simulink model "Roadsense_ScenarioAdapters"  (R2025b)
settings: Solver=FixedStepDiscrete  StartTime=0.0  StopTime=1.0  FixedStep=RsTsBase  RelTol=1e-3
undefined symbols (not defined in the file or in its folder): RsMaxDetections, RsMaxLidarPoints, RsMaxReferencePoints, RsTsBase, RsTsControl, RsTsFusion, RsTsLidarPerception, RsTsPlanning, RsTsSemanticInference
settings Model: DataDictionary=Roadsense_Data.sldd  Creator=ragur  LastModifiedBy=ragur

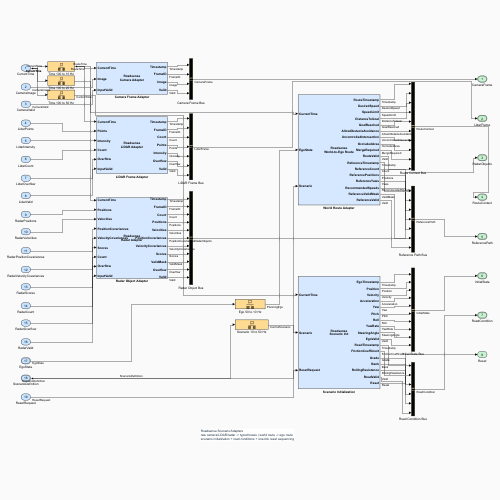
[thumbnail: Simulink's stored preview of the top-level diagram]
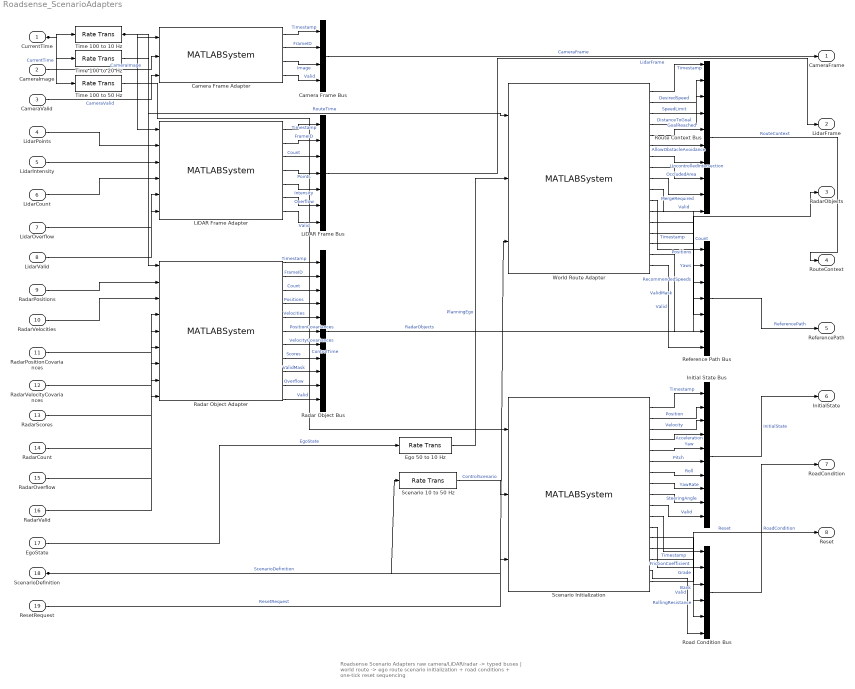
== system Roadsense_ScenarioAdapters ==
  note: Roadsense Scenario Adapters
      | raw camera/LiDAR/radar -> typed buses | world route -> ego route
      | scenario initialization + road conditions + one-tick reset sequencing
  CurrentTime : Inport  OutDataTypeStr=double  PortDimensions=1  SampleTime=RsTsBase
  CameraImage : Inport  Port=2  OutDataTypeStr=uint8  PortDimensions=[480 640 3]  SampleTime=RsTsSemanticInference
  CameraValid : Inport  Port=3  OutDataTypeStr=boolean  PortDimensions=1  SampleTime=RsTsSemanticInference
  LidarPoints : Inport  Port=4  OutDataTypeStr=single  PortDimensions=[120000 3]  SampleTime=RsTsLidarPerception
  LidarIntensity : Inport  Port=5  OutDataTypeStr=single  PortDimensions=[120000 1]  SampleTime=RsTsLidarPerception
  LidarCount : Inport  Port=6  OutDataTypeStr=uint32  PortDimensions=1  SampleTime=RsTsLidarPerception
  LidarOverflow : Inport  Port=7  OutDataTypeStr=boolean  PortDimensions=1  SampleTime=RsTsLidarPerception
  LidarValid : Inport  Port=8  OutDataTypeStr=boolean  PortDimensions=1  SampleTime=RsTsLidarPerception
  RadarPositions : Inport  Port=9  OutDataTypeStr=single  PortDimensions=[256 3]  SampleTime=RsTsFusion
  RadarVelocities : Inport  Port=10  OutDataTypeStr=single  PortDimensions=[256 3]  SampleTime=RsTsFusion
  RadarPositionCovariances : Inport  Port=11  OutDataTypeStr=single  PortDimensions=[3 3 256]  SampleTime=RsTsFusion
  RadarVelocityCovariances : Inport  Port=12  OutDataTypeStr=single  PortDimensions=[3 3 256]  SampleTime=RsTsFusion
  RadarScores : Inport  Port=13  OutDataTypeStr=single  PortDimensions=[256 1]  SampleTime=RsTsFusion
  RadarCount : Inport  Port=14  OutDataTypeStr=uint16  PortDimensions=1  SampleTime=RsTsFusion
  RadarOverflow : Inport  Port=15  OutDataTypeStr=boolean  PortDimensions=1  SampleTime=RsTsFusion
  RadarValid : Inport  Port=16  OutDataTypeStr=boolean  PortDimensions=1  SampleTime=RsTsFusion
  EgoState : Inport  Port=17  OutDataTypeStr=Bus: RsEgoStateBus  PortDimensions=1  SampleTime=RsTsControl
  ScenarioDefinition : Inport  Port=18  OutDataTypeStr=Bus: RsScenarioDefinitionBus  PortDimensions=1  SampleTime=RsTsPlanning
  ResetRequest : Inport  Port=19  OutDataTypeStr=boolean  PortDimensions=1  SampleTime=RsTsControl
  Camera Frame Adapter : MATLABSystem  System=RoadsenseCameraFrameAdapterSystem  SimulateUsing=Code generation
      mask Type: RoadsenseCameraFrameAdapterSystem
  Camera Frame Bus : BusCreator  Inputs=4  OutDataTypeStr=Bus: RsCameraFrameBus
  Ego 50 to 10 Hz : RateTransition  OutPortSampleTime=RsTsPlanning
  Initial State Bus : BusCreator  Inputs=10  OutDataTypeStr=Bus: RsEgoStateBus
  LiDAR Frame Adapter : MATLABSystem  System=RoadsenseLidarFrameAdapterSystem  MaxPoints=double(RsMaxLidarPoints)  SimulateUsing=Code generation
      mask Type: RoadsenseLidarFrameAdapterSystem
  LiDAR Frame Bus : BusCreator  Inputs=7  OutDataTypeStr=Bus: RsLidarFrameBus
  Radar Object Adapter : MATLABSystem  System=RoadsenseRadarObjectAdapterSystem  MaxDetections=double(RsMaxDetections)  SimulateUsing=Code generation
      mask Type: RoadsenseRadarObjectAdapterSystem
  Radar Object Bus : BusCreator  Inputs=11  OutDataTypeStr=Bus: RsRadarObjectListBus
  Reference Path Bus : BusCreator  Inputs=7  OutDataTypeStr=Bus: RsReferencePathBus
  Road Condition Bus : BusCreator  Inputs=6  OutDataTypeStr=Bus: RsRoadConditionBus
  Route Context Bus : BusCreator  Inputs=10  OutDataTypeStr=Bus: RsRouteContextBus
  Scenario 10 to 50 Hz : RateTransition  OutPortSampleTime=RsTsControl
  Scenario Initialization : MATLABSystem  System=RoadsenseScenarioInitializationSystem  SimulateUsing=Code generation
      mask Type: RoadsenseScenarioInitializationSystem
  Time 100 to 10 Hz : RateTransition  OutPortSampleTime=RsTsPlanning
  Time 100 to 20 Hz : RateTransition  OutPortSampleTime=RsTsFusion
  Time 100 to 50 Hz : RateTransition  OutPortSampleTime=RsTsControl
  World Route Adapter : MATLABSystem  System=RoadsenseRouteAdapterSystem  MaxReferencePoints=double(RsMaxReferencePoints)  SimulateUsing=Code generation
      mask Type: RoadsenseRouteAdapterSystem
  CameraFrame : Outport  OutDataTypeStr=Bus: RsCameraFrameBus
  LidarFrame : Outport  Port=2  OutDataTypeStr=Bus: RsLidarFrameBus
  RadarObjects : Outport  Port=3  OutDataTypeStr=Bus: RsRadarObjectListBus
  RouteContext : Outport  Port=4  OutDataTypeStr=Bus: RsRouteContextBus
  ReferencePath : Outport  Port=5  OutDataTypeStr=Bus: RsReferencePathBus
  InitialState : Outport  Port=6  OutDataTypeStr=Bus: RsEgoStateBus
  RoadCondition : Outport  Port=7  OutDataTypeStr=Bus: RsRoadConditionBus
  Reset : Outport  Port=8  OutDataTypeStr=boolean
  wires:
  CurrentTime/1 -> Time 100 to 10 Hz/1, Time 100 to 20 Hz/1, Time 100 to 50 Hz/1  "CurrentTime"
  EgoState/1 -> Ego 50 to 10 Hz/1  "EgoState"
  ScenarioDefinition/1 -> Scenario 10 to 50 Hz/1, World Route Adapter/3  "ScenarioDefinition"
  Time 100 to 10 Hz/1 -> Camera Frame Adapter/1, LiDAR Frame Adapter/1, World Route Adapter/1  "RouteTime"
  CameraImage/1 -> Camera Frame Adapter/2  "CameraImage"
  CameraValid/1 -> Camera Frame Adapter/3  "CameraValid"
  Camera Frame Adapter/1 -> Camera Frame Bus/1  "Timestamp"
  Camera Frame Adapter/2 -> Camera Frame Bus/2  "FrameID"
  Camera Frame Adapter/3 -> Camera Frame Bus/3  "Image"
  Camera Frame Adapter/4 -> Camera Frame Bus/4  "Valid"
  LidarPoints/1 -> LiDAR Frame Adapter/2
  LidarIntensity/1 -> LiDAR Frame Adapter/3
  LidarCount/1 -> LiDAR Frame Adapter/4
  LidarOverflow/1 -> LiDAR Frame Adapter/5
  LidarValid/1 -> LiDAR Frame Adapter/6
  LiDAR Frame Adapter/1 -> LiDAR Frame Bus/1  "Timestamp"
  LiDAR Frame Adapter/2 -> LiDAR Frame Bus/2  "FrameID"
  LiDAR Frame Adapter/3 -> LiDAR Frame Bus/3  "Count"
  LiDAR Frame Adapter/4 -> LiDAR Frame Bus/4  "Points"
  LiDAR Frame Adapter/5 -> LiDAR Frame Bus/5  "Intensity"
  LiDAR Frame Adapter/6 -> LiDAR Frame Bus/6  "Overflow"
  LiDAR Frame Adapter/7 -> LiDAR Frame Bus/7  "Valid"
  Time 100 to 20 Hz/1 -> Radar Object Adapter/1
  RadarPositions/1 -> Radar Object Adapter/2
  RadarVelocities/1 -> Radar Object Adapter/3
  RadarPositionCovariances/1 -> Radar Object Adapter/4
  RadarVelocityCovariances/1 -> Radar Object Adapter/5
  RadarScores/1 -> Radar Object Adapter/6
  RadarCount/1 -> Radar Object Adapter/7
  RadarOverflow/1 -> Radar Object Adapter/8
  RadarValid/1 -> Radar Object Adapter/9
  Radar Object Adapter/1 -> Radar Object Bus/1  "Timestamp"
  Radar Object Adapter/2 -> Radar Object Bus/2  "FrameID"
  Radar Object Adapter/3 -> Radar Object Bus/3  "Count"
  Radar Object Adapter/4 -> Radar Object Bus/4  "Positions"
  Radar Object Adapter/5 -> Radar Object Bus/5  "Velocities"
  Radar Object Adapter/6 -> Radar Object Bus/6  "PositionCovariances"
  Radar Object Adapter/7 -> Radar Object Bus/7  "VelocityCovariances"
  Radar Object Adapter/8 -> Radar Object Bus/8  "Scores"
  Radar Object Adapter/9 -> Radar Object Bus/9  "ValidMask"
  Radar Object Adapter/10 -> Radar Object Bus/10  "Overflow"
  Radar Object Adapter/11 -> Radar Object Bus/11  "Valid"
  Ego 50 to 10 Hz/1 -> World Route Adapter/2  "PlanningEgo"
  World Route Adapter/1 -> Route Context Bus/1  "Timestamp"
  World Route Adapter/2 -> Route Context Bus/2  "DesiredSpeed"
  World Route Adapter/3 -> Route Context Bus/3  "SpeedLimit"
  World Route Adapter/4 -> Route Context Bus/4  "DistanceToGoal"
  World Route Adapter/5 -> Route Context Bus/5  "GoalReached"
  World Route Adapter/6 -> Route Context Bus/6  "AllowObstacleAvoidance"
  World Route Adapter/7 -> Route Context Bus/7  "UncontrolledIntersection"
  World Route Adapter/8 -> Route Context Bus/8  "OccludedArea"
  World Route Adapter/9 -> Route Context Bus/9  "MergeRequired"
  World Route Adapter/10 -> Route Context Bus/10  "Valid"
  World Route Adapter/11 -> Reference Path Bus/1  "Timestamp"
  World Route Adapter/12 -> Reference Path Bus/2  "Count"
  World Route Adapter/13 -> Reference Path Bus/3  "Positions"
  World Route Adapter/14 -> Reference Path Bus/4  "Yaws"
  World Route Adapter/15 -> Reference Path Bus/5  "RecommendedSpeeds"
  World Route Adapter/16 -> Reference Path Bus/6  "ValidMask"
  World Route Adapter/17 -> Reference Path Bus/7  "Valid"
  Time 100 to 50 Hz/1 -> Scenario Initialization/1  "ControlTime"
  Scenario 10 to 50 Hz/1 -> Scenario Initialization/2  "ControlScenario"
  ResetRequest/1 -> Scenario Initialization/3  "ResetRequest"
  Scenario Initialization/1 -> Initial State Bus/1  "Timestamp"
  Scenario Initialization/2 -> Initial State Bus/2  "Position"
  Scenario Initialization/3 -> Initial State Bus/3  "Velocity"
  Scenario Initialization/4 -> Initial State Bus/4  "Acceleration"
  Scenario Initialization/5 -> Initial State Bus/5  "Yaw"
  Scenario Initialization/6 -> Initial State Bus/6  "Pitch"
  Scenario Initialization/7 -> Initial State Bus/7  "Roll"
  Scenario Initialization/8 -> Initial State Bus/8  "YawRate"
  Scenario Initialization/9 -> Initial State Bus/9  "SteeringAngle"
  Scenario Initialization/10 -> Initial State Bus/10  "Valid"
  Scenario Initialization/11 -> Road Condition Bus/1  "Timestamp"
  Scenario Initialization/12 -> Road Condition Bus/2  "FrictionCoefficient"
  Scenario Initialization/13 -> Road Condition Bus/3  "Grade"
  Scenario Initialization/14 -> Road Condition Bus/4  "Bank"
  Scenario Initialization/15 -> Road Condition Bus/5  "RollingResistance"
  Scenario Initialization/16 -> Road Condition Bus/6  "Valid"
  Camera Frame Bus/1 -> CameraFrame/1  "CameraFrame"
  LiDAR Frame Bus/1 -> LidarFrame/1  "LidarFrame"
  Radar Object Bus/1 -> RadarObjects/1  "RadarObjects"
  Route Context Bus/1 -> RouteContext/1  "RouteContext"
  Reference Path Bus/1 -> ReferencePath/1  "ReferencePath"
  Initial State Bus/1 -> InitialState/1  "InitialState"
  Road Condition Bus/1 -> RoadCondition/1  "RoadCondition"
  Scenario Initialization/17 -> Reset/1  "Reset"
